simulink model "rtwdemo_cpp"  (Simulink 7.6)
settings: Solver=FixedStepDiscrete  StartTime=0.0  StopTime=10  FixedStep=1  RelTol=1e-3
libraries: rtwdemowidgets x1
Description:
  | Integrating Arbitrary C++ Code in Simulink(R)
settings Model: Creator=The MathWorks Inc.  ExtModeTrigMode=oneshot  ExtModeArmWhenConnect=off  ExtModeAutoUpdateStatusClock=off
settings MATStruct: SampleTime=1  Offset=0  Priority=[20.0]
settings DataIOCC: LimitDataPoints=off  SaveOutput=off  SignalLogging=off  SaveTime=off  SignalLoggingName=logsOut
settings OptimizationCC: InlineParams=on  InlineInvariantSignals=on  StateBitsets=on  DataBitsets=on  UseTempVars=on  EfficientFloat2IntCast=on  EfficientMapNaN2IntZero=off  BufferReusableBoundary=off
settings DebuggingCC: SolverPrmCheckMsg=none  SigSpecEnsureSampleTimeMsg=none  StrictBusMsg=ErrorOnBusTreatedAsVector
settings HardwareCC: ProdIntDivRoundTo=Zero  ProdEndianess=LittleEndian  ProdHWDeviceType=Generic->32-bit Embedded Processor  TargetHWDeviceType=Generic->32-bit Embedded Processor
settings RTWCC: GenerateReport=on  RTWVerbose=off  ProcessScript=grt_make_rtw_hook  CustomSourceCode="#include \"sfun_cppcount_cpp.h\""  CustomInclude="\"$matlabroot$/simulink/src\""  LaunchReport=on  TargetLang=C++
settings CodeAppCC: ForceParamTrailComments=on
settings GRTTargetCC: TargetFcnLib=ansi_tfl_tmw.mat

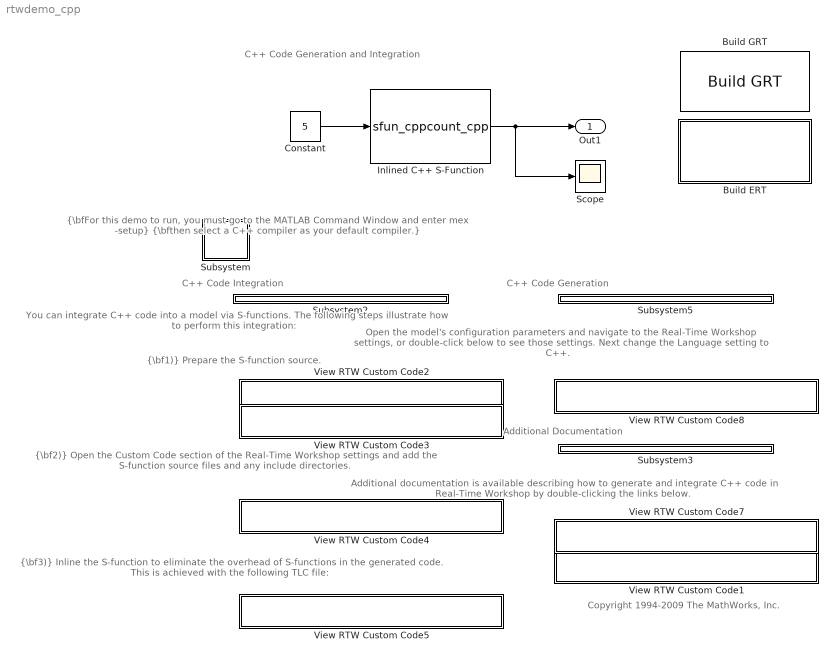
== system rtwdemo_cpp ==
  note: C++ Code Generation and Integration
  note: {\bfFor this demo to run, you must go to the MATLAB Command Window and enter
      |        mex  -setup}
      | {\bfthen select a C++ compiler as your default compiler.}
  note: Additional Documentation
  note: Additional documentation is available
      | describing how to generate and integrate
      | C++ code in Real-Time Workshop by
      | double-clicking the links below.
  note: Open the model's configuration parameters
      | and navigate to the Real-Time Workshop
      | settings, or double-click below to see those
      | settings.  Next change the Language setting
      | to C++.
  note: C++ Code Generation
  note: You can integrate C++ code into a model via
      | S-functions.  The following steps illustrate
      | how to perform this integration:
  note: C++ Code Integration
  note: {\bf2)} Open the Custom Code section of the
      |      Real-Time Workshop settings and add
      |      the S-function source files and any
      |      include directories.
  note: {\bf3)} Inline the S-function to eliminate the
      |        overhead of S-functions in the generated
      |        code.  This is achieved with the following
      |        TLC file:
  note: {\bf1)} Prepare the S-function source.
  note: Copyright 1994-2009 The MathWorks, Inc.
  Build ERT : Subsystem  mask{attrib_overrides={'IncludeMdlTerminateFcn'}}
      mask prompts: attrib_overrides "List of attributes to preserve (cell of strings):"
      mask help: Enter the attributes of the configuration set that you want preserved. Otherwise, the default configuration script will override your current settings.
      settings: OpenFcn=|
      | model=bdroot;
      |                   overrides=get_param(gcb,'attrib_overrides');
      | try
      |   rtwconfiguredemo(model,'noop',false,overrides);
      |   set_param(model,'TargetLang','C++');
      |   rtwbuilddemomodel(model);
      | catch
      |   error(lasterr);
      | end;
      |               clear model overrides;
      mask Display:
      | disp(['Generate Code Using\n',...
      | 	  'Real-Time Workshop\n',...
      | 	  'Embedded Coder\n'...
      | 	  '(double-click)'])
  Build GRT : rtwdemowidgets/Build GRT  SystemSampleTime=-1  attrib_overrides={'InlineParams'}
  Constant : Constant  Value=5  SampleTime=1
  Inlined C++ S-Function : S-Function  FunctionName=sfun_cppcount_cpp  EnableBusSupport=off
      mask Display: disp('Inlined C++\nS-Function');
  Scope : Scope
      settings: TimeRange=10  YMin=0  YMax=60
  Subsystem : Subsystem
      mask init:
      | pos    = get_param(gcb, 'Position');
      | width  = pos(3) - pos(1);
      | height = pos(4) - pos(2);
      | 
      | marginPercent = 20;
      | marginPixels  = round(marginPercent / 100 * width);
      | 
      | x1 = width - marginPixels;
      | y1 = height;
      | x2 = width;
      | y2 = height - marginPixels;
      | x3 = width;
      | y3 = marginPixels;
      | x4 = width - marginPixels;
      | y4 = 0;
      | x5 = marginPixels;
      | y5 = 0;
      | x6 = 0;
      | y6 = marginPixels;
      | x7 = 0;
      | y7 = height - marginPixels;
      | x8 = marginPixels;
      | y8 = height;
      | 
      | xvec = [x1, x2, x3, x4, x5, x6, x7, x8];
      | yvec = [y1, y2, y3, y4, y5, y6, y7, y8];
      mask Display:
      | color('red');
      | patch(xvec, yvec);
      | color('white');
      | disp('!');
  Subsystem2 : Subsystem
  Subsystem3 : Subsystem
  Subsystem5 : Subsystem
  View RTW Custom Code1 : Subsystem
      mask init:
      | pos    = get_param(gcb, 'Position');
      | width  = pos(3) - pos(1);
      | height = pos(4) - pos(2);
      | 
      | 
      | % Compute arrow coordinates
      | arrowW = width  / 20;
      | arrowH = height / 2.5;
      | arrowX = width  / 50;
      | arrowY = height / 3;
      | arrowXvec = [arrowX, arrowX, arrowX + arrowW];
      | arrowYvec = [arrowY, arrowY + arrowH, arrowY + arrowH / 2];
      | 
      | % Compute text position
      | textXbuff = width / 30;
      | textX  = arrowX + arrowW + textXbuff;
      | textY  = height / 2;
      settings: OpenFcn=helpview([docroot '/toolbox/rtw/helptargets.map'], 'rtw_cpp_limitations')
      mask Display:
      | patch(arrowXvec, arrowYvec);
      | text(textX, textY, 'C++ Limitations');
  View RTW Custom Code2 : Subsystem
      mask init: same as rtwdemo_cpp/View RTW Custom Code1
      settings: OpenFcn=|
      | filename=fullfile(matlabroot, 'simulink', 'src', 'sfun_cppcount_cpp.cpp');
      | eval('edit(filename)'); clear filename;
      mask Display:
      | patch(arrowXvec, arrowYvec);
      | text(textX, textY, 'Open sfun_cppcount_cpp.cpp');
  View RTW Custom Code3 : Subsystem
      mask init: same as rtwdemo_cpp/View RTW Custom Code1
      settings: OpenFcn=|
      | filename=fullfile(matlabroot, 'simulink', 'src', 'sfun_cppcount_cpp.h');
      | eval('edit(filename)');  clear filename;
      mask Display:
      | patch(arrowXvec, arrowYvec);
      | text(textX, textY, 'Open sfun_cppcount_cpp.h');
  View RTW Custom Code4 : Subsystem
      mask init: same as rtwdemo_cpp/View RTW Custom Code1
      settings: OpenFcn=|
      | model = bdroot;
      | dlg = slCfgPrmDlg(model,'Open');
      | dlg = slCfgPrmDlg(bdroot,'TurnToPage','Real-Time Workshop/Custom Code');
      | clear model dlg;
      mask Display:
      | patch(arrowXvec, arrowYvec);
      | text(textX, textY, 'Open Custom Code Settings');
  View RTW Custom Code5 : Subsystem
      mask init: same as rtwdemo_cpp/View RTW Custom Code1
      settings: OpenFcn=|
      | filename=fullfile(matlabroot, 'toolbox','simulink', 'blocks', 'tlc_c','sfun_cppcount_cpp.tlc');
      | eval('edit(filename)');                            clear filename;
      mask Display:
      | patch(arrowXvec, arrowYvec);
      | text(textX, textY, 'Open sfun_cppcount_cpp.tlc');
  View RTW Custom Code7 : Subsystem
      mask init: same as rtwdemo_cpp/View RTW Custom Code1
      settings: OpenFcn=helpview([docroot '/toolbox/rtw/helptargets.map'], 'rtw_language_support')
      mask Display:
      | patch(arrowXvec, arrowYvec);
      | text(textX, textY, 'C++ Documentation');
  View RTW Custom Code8 : Subsystem
      mask init: same as rtwdemo_cpp/View RTW Custom Code1
      settings: OpenFcn=|
      | model = bdroot;
      | dlg = slCfgPrmDlg(model,'Open');
      | dlg = slCfgPrmDlg(bdroot,'TurnToPage','Real-Time Workshop');
      | clear model dlg;
      mask Display:
      | patch(arrowXvec, arrowYvec);
      | text(textX, textY, 'Open Real-Time Workshop Settings');
  Out1 : Outport
  wires:
  Inlined C++ S-Function/1 -> Out1/1, Scope/1
  Constant/1 -> Inlined C++ S-Function/1

== system rtwdemo_cpp/Build ERT ==

== system rtwdemo_cpp/Subsystem ==

== system rtwdemo_cpp/Subsystem2 ==

== system rtwdemo_cpp/Subsystem3 ==

== system rtwdemo_cpp/Subsystem5 ==

== system rtwdemo_cpp/View RTW Custom Code1 ==

== system rtwdemo_cpp/View RTW Custom Code2 ==

== system rtwdemo_cpp/View RTW Custom Code3 ==

== system rtwdemo_cpp/View RTW Custom Code4 ==

== system rtwdemo_cpp/View RTW Custom Code5 ==

== system rtwdemo_cpp/View RTW Custom Code7 ==

== system rtwdemo_cpp/View RTW Custom Code8 ==
